simulink model "Q1_dynamic_suspention_Vehical"  (R2024b)
settings: Solver=VariableStepAuto  StartTime=0.0  StopTime=15  RelTol=1e-3
model workspace (MAT data in the model file):
  C_d = 1
  C_s = 2
  M = 1
settings Model: Creator=chall  LastModifiedBy=chall

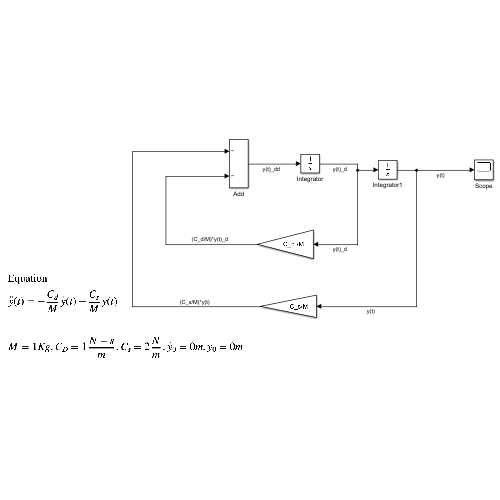
[thumbnail: Simulink's stored preview of the top-level diagram]
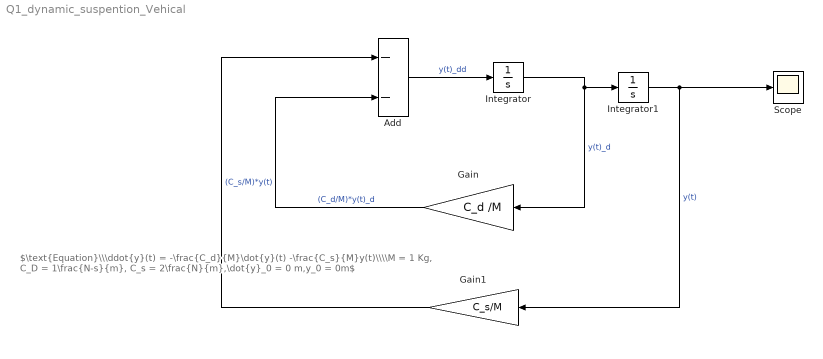
== system Q1_dynamic_suspention_Vehical ==
  note: $\text{Equation}\\\ddot{y}(t) = -\frac{C_d}{M}\dot{y}(t) -\frac{C_s}{M}y(t)\\\\M = 1 Kg, C_D = 1\frac{N-s}{m}, C_s = 2\frac{N}{m},\dot{y}_0 = 0 m,y_0 = 0m$
  Add : Sum  Inputs=--
  Gain : Gain  Gain=C_d /M
  Gain1 : Gain  Gain=C_s/M
  Integrator : Integrator
  Integrator1 : Integrator
  Scope : Scope
  wires:
  Add/1 -> Integrator/1  "y(t)_dd"
  Integrator/1 -> Gain/1, Integrator1/1  "y(t)_d"
  Integrator1/1 -> Gain1/1, Scope/1  "y(t)"
  Gain/1 -> Add/2  "(C_d/M)*y(t)_d"
  Gain1/1 -> Add/1  "(C_s/M)*y(t)"
